simulink model "rtsiggen"  (Simulink 6.0)
settings: Solver=ode4  StartTime=0.0  StopTime=10.0  RelTol=1e-3
libraries: rtwinlib x1
settings Model: Creator=Houska  LastModifiedBy=Houska  ExtModeMexFile=rtwinext  ExtModeTrigType=signal  ExtModeTrigLevel=0.500000  ProdHWDeviceType=32-bit Real-Time Windows Target
settings ConfigSet: SimulationMode=external
settings DataIOCC: SaveOutput=off  SaveTime=off  SignalLoggingName=logsOut
settings OptimizationCC: MultiInstanced=off
settings FormatCC: IgnoreBidirectionalLines=off
settings HardwareCC: ProdIntDivRoundTo=Zero  ProdEndianess=LittleEndian  ProdHWDeviceType=32-bit Real-Time Windows Target
settings RTWCC: SystemTargetFile=rtwin.tlc  TemplateMakefile=rtwin.tmf  Description=Real-Time Windows Target  ProcessScript=rtwin_make_rtw_hook
settings CodeAppCC: SimulinkBlockComments=off
settings RTWinTargetCC: TargetFcnLib=iso_c_tmw.mat  CCOptimize=on

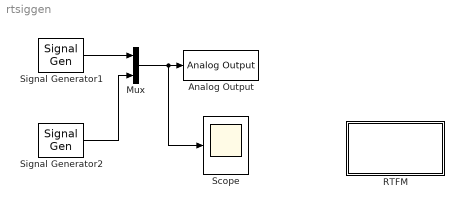
== system rtsiggen ==
  Analog Output : rtwinlib/Analog Output  SampleTime=1e-3  DrvAddress=0  DrvOptions=0  Channels=1:2  RangeMode=1  VoltRange=1  InitialValue=[]  FinalValue=[]
  Mux : Mux  Inputs=2
  "RTFM " : Subsystem
      mask Type: Frame-Based Simulation Info
      mask Display: disp('Info')
  Scope : Scope
      settings: TimeRange=1  YMin=-2.11111  YMax=2.17647  DataFormat=Structure
  Signal Generator1 : SignalGenerator  Amplitude=1.000000  Frequency=5
  Signal Generator2 : SignalGenerator  WaveForm=square  Amplitude=0.25000000  Frequency=2.500000
  wires:
  Signal Generator2/1 -> Mux/2
  Signal Generator1/1 -> Mux/1
  Mux/1 -> Scope/1, Analog Output/1

== system rtsiggen/RTFM  ==
  note: How to run this demo:
      |
      | 1) Open the Analog Output block and select your data acquisition board.
      |      If there's no board installed, install it using the Install new board button.
      | 2) Build the model using Tools->Real-Time Workshop->Build Model.
      | 3) Connect to the real-time code using Simulation->Connect to target.
      | 4) Start the real-time execution using Simulation->Start real-time code.
      |
      | Note: To run this demo, you must have a data acquisition board plugged into
      | your computer.
